simulink library "athenaControls"  (R2018b)
settings: Solver=VariableStepAuto  StartTime=0.0  StopTime=10.0  RelTol=1e-3
settings Model: Creator=rmathijn  LastModifiedBy=rmathijn

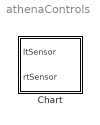
== system athenaControls ==
  Chart : Stateflow chart  TreatAsAtomicUnit=on

== stateflow chart athenaControls/Chart ==
  state Controls
    state LSHold
    state NoChange
      exit:
      send(BUTTON_ACTIVITY, Drive)
    state RSHold
    state ShortPress
    state LongPress
    (default) -> NoChange
    NoChange -> LSHold [order 2] : [ltSensor == 1 && rtSensor == 0]
        | {send(LHOLD, Drive)}
    NoChange -> RSHold [order 3] : [ltSensor == 0 && rtSensor == 1]
        | {send(RHOLD, Drive)}
    RSHold -> NoChange : [rtSensor == 0 && ltSensor == 0]
        | {send(RELEASE, Drive)}
    LSHold -> NoChange : [ltSensor == 0 && rtSensor == 0]
        | {send(RELEASE, Drive)}
    NoChange -> ShortPress [order 1] : [ltSensor == 1 && rtSensor == 1]
    ShortPress -> NoChange [order 2] : [ltSensor == 0 && rtSensor == 0]
        | {send(SHORT_PRESS, Drive)}
    LongPress -> NoChange : [ltSensor == 0 && rtSensor == 0]
        | {send(LONG_PRESS, Drive)}
    ShortPress -> LongPress [order 1] : [after(1,sec)]
  data: ltSensor input; rtSensor input
  events: LHOLD local FUNCTION_CALL_EVENT; LONG_PRESS local FUNCTION_CALL_EVENT; RELEASE local FUNCTION_CALL_EVENT; RHOLD local FUNCTION_CALL_EVENT; SHORT_PRESS local FUNCTION_CALL_EVENT; BUTTON_ACTIVITY local FUNCTION_CALL_EVENT
